simulink model "Lab07B"  (R2021a)
settings: Solver=VariableStepAuto  StartTime=0.0  StopTime=10.0  RelTol=1e-3
undefined symbols (not defined in the file): DiscIntNeverNeededParam
libraries: dsparch4 x1, commsynccomp2 x1
settings Model: Creator=shirs  LastModifiedBy=shirs

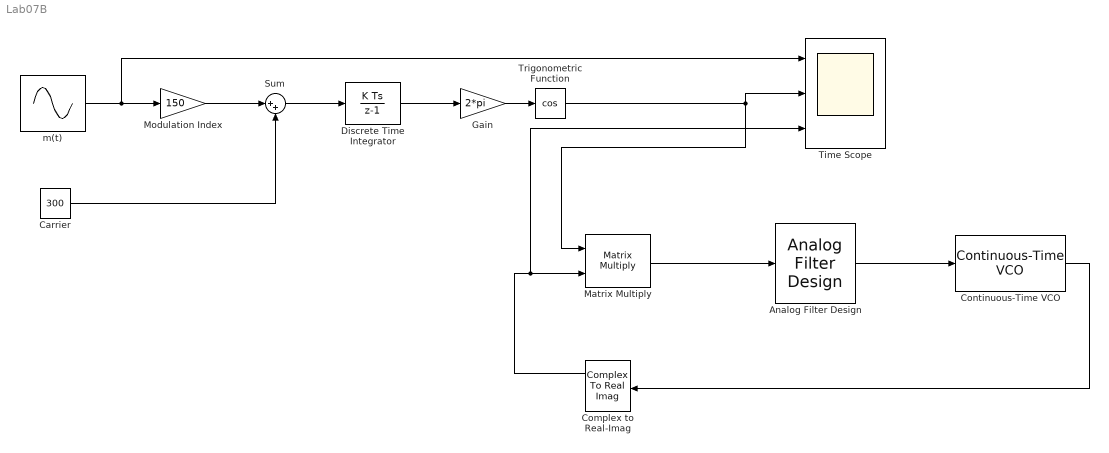
== system Lab07B ==
  Analog Filter Design : dsparch4/Analog Filter Design  method=Butterworth  filttype=Lowpass  N=10  Wlo=2*pi*10  Whi=80  Rp=2  Rs=40
  Carrier : Constant  Value=300
  Complex to Real-Imag : ComplexToRealImag
  Continuous-Time VCO : commsynccomp2/Continuous-Time VCO  Ac=1  Fc=10  Kc=50  Ph=0
      settings: SourceProductBaseCode=CM
  Discrete Time Integrator : DiscreteIntegrator  SampleTime=1/98000  ICPrevOutput=DiscIntNeverNeededParam  ICPrevScaledInput=DiscIntNeverNeededParam
  Gain : Gain  Gain=2*pi
  Matrix Multiply : Product  Multiplication=Matrix(*)
  Modulation Index : Gain  Gain=150
  Sum : Sum  Inputs=|++
  Time Scope : Scope  NumInputPorts=3
  Trigonometric Function : Trigonometry  Operator=cos
  m(t) : Sin  Frequency=10  Phase=90  SampleTime=1/98000
  wires:
  Sum/1 -> Discrete Time Integrator/1
  Discrete Time Integrator/1 -> Gain/1
  Gain/1 -> Trigonometric Function/1
  Modulation Index/1 -> Sum/1
  m(t)/1 -> Time Scope/1, Modulation Index/1
  Carrier/1 -> Sum/2
  Matrix Multiply/1 -> Analog Filter Design/1
  Analog Filter Design/1 -> Continuous-Time VCO/1
  Continuous-Time VCO/1 -> Complex to Real-Imag/1
  Complex to Real-Imag/1 -> Time Scope/3, Matrix Multiply/2
  Trigonometric Function/1 -> Time Scope/2, Matrix Multiply/1
